simulink model "control"  (R2018b)
settings: Solver=VariableStepAuto  StartTime=0.0  StopTime=80  RelTol=1e-3
values from neighbouring files (symbols this model uses):
  a = sqrt(2*b)    [bilateral_control_parameters.m]
  b = 20    [bilateral_control_parameters.m]
  Bm = 20    [bilateral_control_parameters.m]
  Gf = 1    [bilateral_control_parameters.m]
  ke = 100    [bilateral_control_parameters.m]
  kh = 10000    [bilateral_control_parameters.m]
  m = 1    [bilateral_control_parameters.m]
  td = 0.1    [bilateral_control_parameters.m]
settings Model: Creator=Bibiana  LastModifiedBy=mariorc
settings DebuggingCC: LibraryContextMissingDiagnostic=none
settings SFSimCC: SimUseLocalCustomCode=off
settings RTWCC: RTWUseLocalCustomCode=off

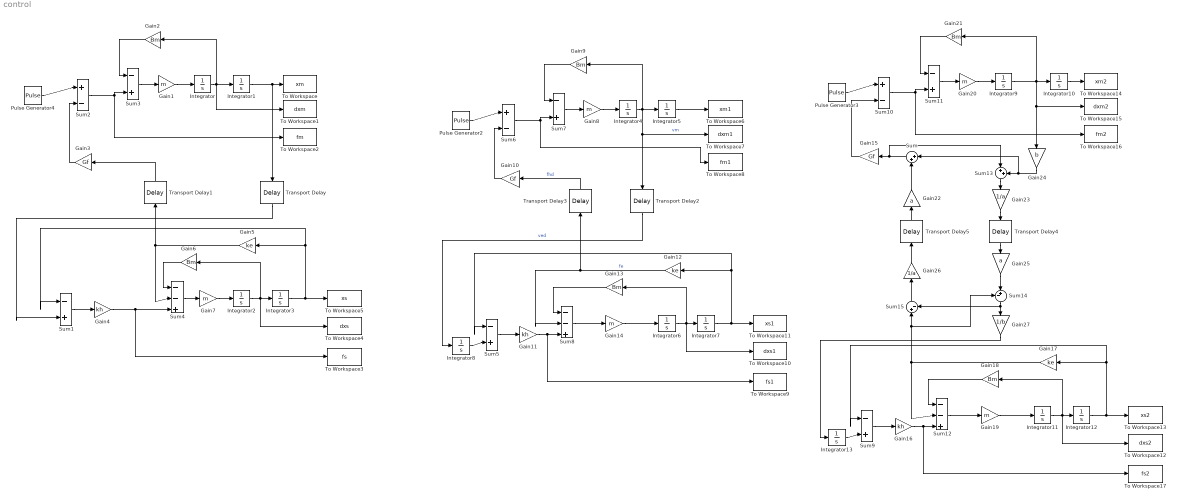
== system control ==
  Gain{1,7..8,14,19..20} (6 alike) : Gain  Gain=m
  Gain10 : Gain  Gain=Gf
  Gain11 : Gain  Gain=kh
  Gain12 : Gain  Gain=ke
  Gain{2,6,9,13,18,21} (6 alike) : Gain  Gain=Bm
  Gain15 : Gain  Gain=Gf
  Gain16 : Gain  Gain=kh
  Gain17 : Gain  Gain=ke
  Gain22 : Gain  Gain=a
  Gain23 : Gain  Gain=1/a
  Gain24 : Gain  Gain=b
  Gain25 : Gain  Gain=a
  Gain26 : Gain  Gain=1/a
  Gain27 : Gain  Gain=1/b
  Gain3 : Gain  Gain=Gf
  Gain4 : Gain  Gain=kh
  Gain5 : Gain  Gain=ke
  Integrator{,1..13} (14 alike) : Integrator
  Pulse Generator2 : DiscretePulseGenerator  PulseType=Time based  Period=40  PulseWidth=50
  Pulse Generator3 : DiscretePulseGenerator  PulseType=Time based  Period=40  PulseWidth=50
  Pulse Generator4 : DiscretePulseGenerator  PulseType=Time based  Period=40  PulseWidth=50  VectorParams1D=off
  Sum : Sum  Inputs=|++
  Sum{1,3,5,7,9,11} (6 alike) : Sum  Inputs=|-+
  Sum{2,6,10,15} (4 alike) : Sum  Inputs=|+-
  Sum12 : Sum  Inputs=|--+
  Sum13 : Sum  Inputs=|++
  Sum14 : Sum  Inputs=-+|
  Sum4 : Sum  Inputs=|--+
  Sum8 : Sum  Inputs=|--+
  To Workspace : ToWorkspace  VariableName=xm  SaveFormat=Timeseries  SampleTime=-1
  To Workspace1 : ToWorkspace  VariableName=dxm  SaveFormat=Timeseries  SampleTime=-1
  To Workspace10 : ToWorkspace  VariableName=dxs1  SaveFormat=Timeseries  SampleTime=-1
  To Workspace11 : ToWorkspace  VariableName=xs1  SaveFormat=Timeseries  SampleTime=-1
  To Workspace12 : ToWorkspace  VariableName=dxs2  SaveFormat=Timeseries  SampleTime=-1
  To Workspace13 : ToWorkspace  VariableName=xs2  SaveFormat=Timeseries  SampleTime=-1
  To Workspace14 : ToWorkspace  VariableName=xm2  SaveFormat=Timeseries  SampleTime=-1
  To Workspace15 : ToWorkspace  VariableName=dxm2  SaveFormat=Timeseries  SampleTime=-1
  To Workspace16 : ToWorkspace  VariableName=fm2  SaveFormat=Timeseries  SampleTime=-1
  To Workspace17 : ToWorkspace  VariableName=fs2  SaveFormat=Timeseries  SampleTime=-1
  To Workspace2 : ToWorkspace  VariableName=fm  SaveFormat=Timeseries  SampleTime=-1
  To Workspace3 : ToWorkspace  VariableName=fs  SaveFormat=Timeseries  SampleTime=-1
  To Workspace4 : ToWorkspace  VariableName=dxs  SaveFormat=Timeseries  SampleTime=-1
  To Workspace5 : ToWorkspace  VariableName=xs  SaveFormat=Timeseries  SampleTime=-1
  To Workspace6 : ToWorkspace  VariableName=xm1  SaveFormat=Timeseries  SampleTime=-1
  To Workspace7 : ToWorkspace  VariableName=dxm1  SaveFormat=Timeseries  SampleTime=-1
  To Workspace8 : ToWorkspace  VariableName=fm1  SaveFormat=Timeseries  SampleTime=-1
  To Workspace9 : ToWorkspace  VariableName=fs1  SaveFormat=Timeseries  SampleTime=-1
  Transport Delay{,1..5} (6 alike) : TransportDelay  DelayTime=td
  wires:
  Sum2/1 -> To Workspace2/1, Sum3/2
  Pulse Generator4/1 -> Sum2/1
  Gain2/1 -> Sum3/1
  Sum3/1 -> Gain1/1
  Integrator/1 -> To Workspace1/1, Gain2/1, Integrator1/1
  Gain1/1 -> Integrator/1
  Integrator1/1 -> Transport Delay/1, To Workspace/1
  Gain3/1 -> Sum2/2
  Transport Delay1/1 -> Gain3/1
  Sum1/1 -> Gain4/1
  Transport Delay/1 -> Sum1/2
  Integrator2/1 -> To Workspace4/1, Gain6/1, Integrator3/1
  Gain7/1 -> Integrator2/1
  Gain6/1 -> Sum4/1
  Sum4/1 -> Gain7/1
  Gain5/1 -> Transport Delay1/1, Sum4/2
  Gain4/1 -> To Workspace3/1, Sum4/3
  Integrator3/1 -> Gain5/1, Sum1/1, To Workspace5/1
  Gain11/1 -> To Workspace9/1, Sum8/3
  Integrator7/1 -> Gain12/1, Sum5/1, To Workspace11/1
  Sum5/1 -> Gain11/1
  Sum8/1 -> Gain14/1
  Integrator6/1 -> To Workspace10/1, Gain13/1, Integrator7/1
  Integrator5/1 -> To Workspace6/1
  Gain12/1 -> Sum8/2, Transport Delay3/1  "fe"
  Gain13/1 -> Sum8/1
  Gain10/1 -> Sum6/2
  Transport Delay2/1 -> Integrator8/1  "ved"
  Gain8/1 -> Integrator4/1
  Transport Delay3/1 -> Gain10/1  "fhd"
  Sum7/1 -> Gain8/1
  Gain14/1 -> Integrator6/1
  Integrator4/1 -> To Workspace7/1, Transport Delay2/1, Gain9/1, Integrator5/1  "vm"
  Sum6/1 -> To Workspace8/1, Sum7/2
  Pulse Generator2/1 -> Sum6/1
  Gain9/1 -> Sum7/1
  Integrator8/1 -> Sum5/2
  Gain21/1 -> Sum11/1
  Pulse Generator3/1 -> Sum10/1
  Integrator9/1 -> Gain21/1, Gain24/1, To Workspace15/1, Integrator10/1
  Sum10/1 -> To Workspace16/1, Sum11/2
  Integrator10/1 -> To Workspace14/1
  Gain18/1 -> Sum12/1
  Gain20/1 -> Integrator9/1
  Sum11/1 -> Gain20/1
  Gain15/1 -> Sum10/2
  Integrator12/1 -> Gain17/1, Sum9/1, To Workspace13/1
  Gain19/1 -> Integrator11/1
  Integrator13/1 -> Sum9/2
  Integrator11/1 -> To Workspace12/1, Gain18/1, Integrator12/1
  Sum12/1 -> Gain19/1
  Sum9/1 -> Gain16/1
  Gain16/1 -> To Workspace17/1, Sum12/3
  Gain17/1 -> Sum12/2, Sum14/1, Sum15/1
  Sum/1 -> Sum13/1, Gain15/1
  Transport Delay5/1 -> Gain22/1
  Gain22/1 -> Sum/2
  Sum13/1 -> Gain23/1
  Gain24/1 -> Sum13/2, Sum/1
  Gain26/1 -> Transport Delay5/1
  Gain25/1 -> Sum14/2
  Sum14/1 -> Sum15/2, Gain27/1
  Gain27/1 -> Integrator13/1
  Sum15/1 -> Gain26/1
  Transport Delay4/1 -> Gain25/1
  Gain23/1 -> Transport Delay4/1
